simulink model "Type1_b"  (R2019a)
settings: Solver=VariableStepAuto  StartTime=0.0  StopTime=10  RelTol=1e-3
libraries: simulink x2
settings Model: Creator=admin  LastModifiedBy=admin

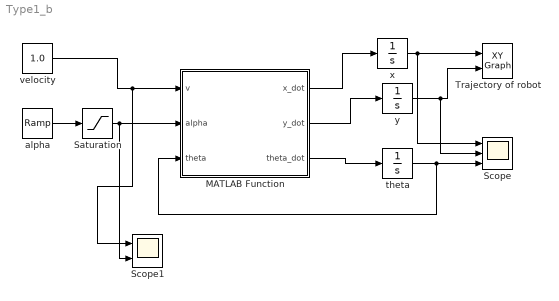
== system Type1_b ==
  MATLAB Function : MATLAB Function  TreatAsAtomicUnit=on
  Saturation : Saturate  UpperLimit=pi/4  LowerLimit=-pi/4
  Scope : Scope  NumInputPorts=3
  Scope1 : Scope  NumInputPorts=2
  Trajectory of robot : simulink/Sinks/XY Graph  xmin=-1  xmax=5  ymin=-1  ymax=7  st=-1
  alpha : simulink/Sources/Ramp  slope=0.4  start=0  InitialOutput=0
  theta : Integrator
  velocity : Constant  Value=1.0
  x : Integrator
  y : Integrator
  wires:
  velocity/1 -> Scope1/1, MATLAB Function/1(v)
  alpha/1 -> Saturation/1
  Saturation/1 -> Scope1/2, MATLAB Function/2(alpha)
  MATLAB Function/2(y_dot) -> y/1
  MATLAB Function/3(theta_dot) -> theta/1
  MATLAB Function/1(x_dot) -> x/1
  y/1 -> Scope/2, Trajectory of robot/2
  theta/1 -> MATLAB Function/3(theta), Scope/3
  x/1 -> Scope/1, Trajectory of robot/1

== matlab function Type1_b/MATLAB Function ==
  data: v input; x_dot output; alpha input; y_dot output; theta_dot output; theta input
function [x_dot, y_dot, theta_dot] = tricycle_type_1(v, alpha,theta)
d = sqrt(3.1)
x_dot = v*cos(alpha)*cos(theta);
y_dot = v*cos(alpha)*sin(theta);
theta_dot = v/d*sin(alpha);
